simulink model "cic5jie"  (R2013a)
settings: Solver=ode45  StartTime=0.0  StopTime=1000  RelTol=1e-3
libraries: dspsigops x1
settings Model: Creator=Administrator  LastModifiedBy=Administrator

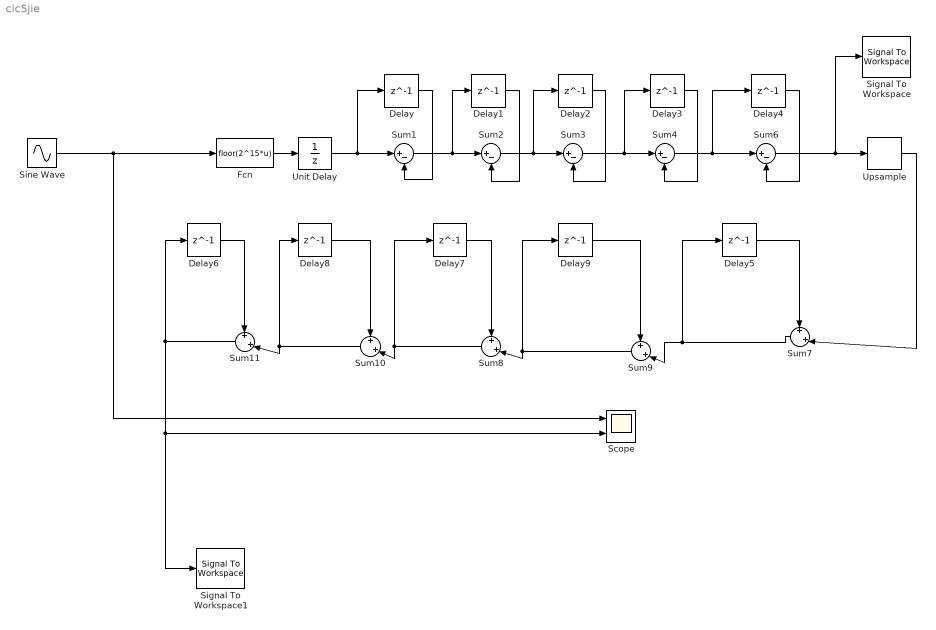
== system cic5jie ==
  Delay{,1..9} (10 alike) : Delay  DelayLength=1  InitialCondition=0
  Fcn : Fcn  Expr=floor(2^15*u)
  Scope : Scope  NumInputPorts=2
      settings: YMin=-5~-5  YMax=5~5
  Signal To Workspace : SignalToWorkspace  VariableName=yout
      settings: CopyFcn=dspblkcopystw(gcbh);
  Signal To Workspace1 : SignalToWorkspace  VariableName=yout1
      settings: CopyFcn=dspblkcopystw(gcbh);
  Sine Wave : Sin  Frequency=10  SampleTime=8
  Sum{1..4,6} (5 alike) : Sum  Inputs=|+-
  Sum{7..11} (5 alike) : Sum  Inputs=+|+|
  Unit Delay : UnitDelay  SampleTime=-1
  Upsample : dspsigops/Upsample  N=8  phase=0  InputProcessing=Columns as channels (frame based)  RateOptions=Allow multirate processing  ic=0  mode=Unused parameter value
  wires:
  Sine Wave/1 -> Fcn/1, Scope/1
  Fcn/1 -> Unit Delay/1
  Unit Delay/1 -> Sum1/1, Delay/1
  Delay/1 -> Sum1/2
  Sum1/1 -> Delay1/1, Sum2/1
  Delay1/1 -> Sum2/2
  Sum2/1 -> Delay2/1, Sum3/1
  Delay2/1 -> Sum3/2
  Sum3/1 -> Delay3/1, Sum4/1
  Delay3/1 -> Sum4/2
  Sum4/1 -> Delay4/1, Sum6/1
  Delay4/1 -> Sum6/2
  Delay5/1 -> Sum7/1
  Sum7/1 -> Delay5/1, Sum9/2
  Delay9/1 -> Sum9/1
  Sum9/1 -> Delay9/1, Sum8/2
  Delay7/1 -> Sum8/1
  Sum8/1 -> Delay7/1, Sum10/2
  Delay8/1 -> Sum10/1
  Sum10/1 -> Delay8/1, Sum11/2
  Delay6/1 -> Sum11/1
  Sum11/1 -> Delay6/1, Signal To Workspace1/1, Scope/2
  Sum6/1 -> Signal To Workspace/1, Upsample/1
  Upsample/1 -> Sum7/2
